simulink model "sgMdl_IO781_AFDXLoopback"  (R2024b)
settings: Solver=FixedStepAuto  StartTime=0.0  StopTime=inf  RelTol=1e-3  EnableMultiTasking=on
libraries: slrealtimeutilitieslib x4, speedgoatlib_IO781 x3, simulink x1
Description:
  | IO781 - AFDX Loopback
settings Model: sg_rtwmakecfg_data=_sg_IO75X_v1_2_0__a664api_  ModifiedByFormat=Speedgoat  SimulationMode=external  ExtModeTrigDuration=100000  Creator=Speedgoat  LastModifiedBy=Speedgoat
settings SolverCC: ConcurrentTasks=on  AlgebraicLoopSolver=TrustRegion  PositivePriorityOrder=on
settings DataIOCC: LimitDataPoints=on  SaveFormat=Array  ReturnWorkspaceOutputs=off
settings OptimizationCC: BlockReduction=off  OptimizeBlockIOStorage=off  BufferReuse=off  GlobalBufferReuse=off  ExpressionFolding=off  LocalBlockOutputs=off
settings DebuggingCC: UnderspecifiedInitializationDetection=Classic  MergeDetectMultiDrivingBlocksExec=none  SolverPrmCheckMsg=warning  TasksWithSamePriorityMsg=none  UnconnectedInputMsg=warning  UnconnectedOutputMsg=warning  UnconnectedLineMsg=warning  SFUnexpectedBacktrackingDiag=warning  SFNoUnconditionalDefaultTransitionDiag=warning  ArithmeticOperatorsInVariantConditions=warning
settings HardwareCC: ProdBitPerLong=64  ProdLongLongMode=on  ProdHWDeviceType=Intel->x86-64 (Linux 64)
settings ModelReferenceCC: EnableRefExpFcnMdlSchedulingChecks=on  PropagateSignalLabelsOutOfModel=off
settings SFSimCC: SimUseLocalCustomCode=off  CustomCodeUndefinedFunction=UseInterfaceOnly
settings RTWCC: Description=Speedgoat Real-Time Target Machine  SystemTargetFile=speedgoat.tlc  TemplateMakefile=slrealtime_default_tmf  RTWUseLocalCustomCode=off  Toolchain=Simulink Real-Time Toolchain  BuildConfiguration=Faster Runs  TargetLang=C++  GPUComputeCapability=3.5  DLArmComputeVersion=19.05
settings CodeAppCC: StateflowObjectComments=on
settings SimulinkRealTimeTargetCC: SubcomponentCodeInterfacePackaging=Reusable function  InstructionSetFMA=off  LogToMDFFile=off  SLRTFileLogMaxRuns=10  UseGCCFastMath=on
settings ConfigComp: CovMetricSettings=dw  CovSaveCumulativeToWorkspaceVar=on  CovSaveSingleToWorkspaceVar=on  CovExternalEMLEnable=off  CovSFcnEnable=off  CovBoundaryAbsTol=1.0e-5

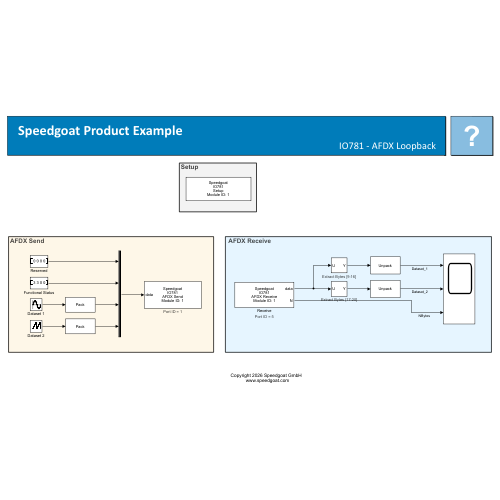
[thumbnail: Simulink's stored preview of the top-level diagram]
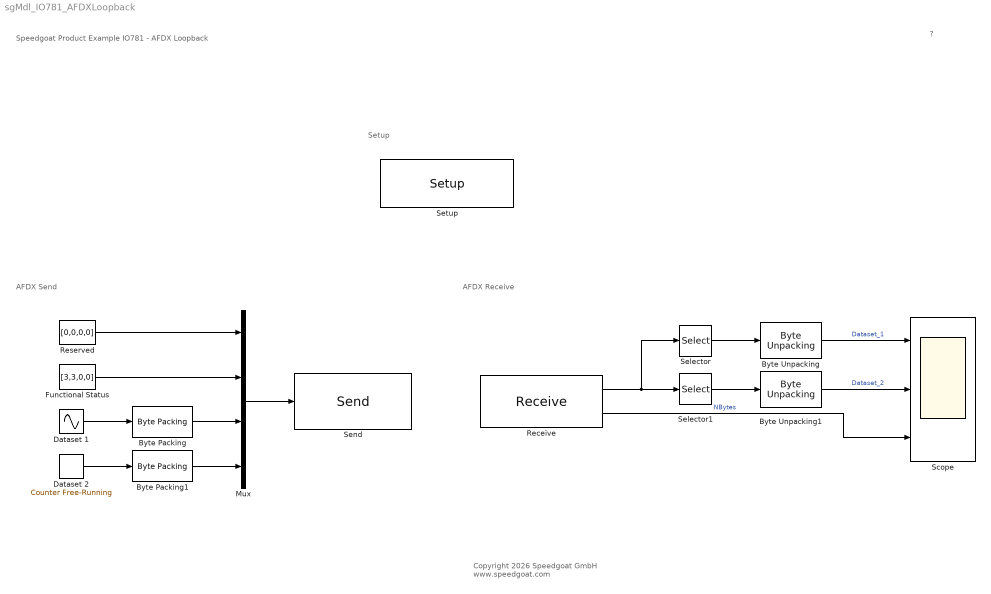
== system sgMdl_IO781_AFDXLoopback ==
  note: Setup
  note: AFDX Send
  note: AFDX Receive
  note: Speedgoat Product Example
      | IO781 - AFDX Loopback
  note: ?
  note: Copyright 2026 Speedgoat GmbH
      |  www.speedgoat.com
  Byte Packing : slrealtimeutilitieslib/Byte Packing  MaskPackedDataType=uint8  MaskUnpackedDataTypes={'double'}  MaskAlignment=1
  Byte Packing1 : slrealtimeutilitieslib/Byte Packing  MaskPackedDataType=uint8  MaskUnpackedDataTypes={'uint32'}  MaskAlignment=1
  Byte Unpacking : slrealtimeutilitieslib/Byte Unpacking  MaskUnpackedDataTypes={'double'}  MaskUnpackedDataSizes={[1]}  MaskAlignment=1
  Byte Unpacking1 : slrealtimeutilitieslib/Byte Unpacking  MaskUnpackedDataTypes={'uint32'}  MaskUnpackedDataSizes={[1]}  MaskAlignment=1
  Dataset 1 : Sin  Amplitude=50  Frequency=2*pi  SampleTime=0.01
  Dataset 2 : simulink/Sources/Counter Free-Running  NumBits=32  tsamp=0.01
  Functional Status : Constant  Value=[3,3,0,0]  OutDataTypeStr=uint8  SampleTime=0.01
  Mux : Mux
  Receive : speedgoatlib_IO781/Receive   parModuleId=1  parSampleTime=0.01  parPortId=5  parRxMsgLen=20
      settings: AttributesFormatString=Port ID = %<parPortId>  SourceProductName=Simulink Real-Time: Speedgoat Library
  "Reserved " : Constant  Value=[0,0,0,0]  OutDataTypeStr=uint8  SampleTime=0.01
  Scope : Scope  NumInputPorts=3
  Selector : Selector  InputPortWidth=20  IndexOptions=Index vector (dialog)  Indices=[9:16]  OutputSizes=1
      settings: AttributesFormatString=Extract Bytes %<Indices>
  Selector1 : Selector  InputPortWidth=20  IndexOptions=Index vector (dialog)  Indices=[17:20]  OutputSizes=1
      settings: AttributesFormatString=Extract Bytes %<Indices>
  "Send " : speedgoatlib_IO781/Send   parModuleId=1  parSampleTime=-1  parPortId=1  parTxMsgLen=20
      settings: AttributesFormatString=Port ID = %<parPortId>  SourceProductName=Simulink Real-Time: Speedgoat Library
  "Setup " : speedgoatlib_IO781/Setup   parModuleId=1  parConfigFile='IO781_Config.adc'
      settings: SourceProductName=Simulink Real-Time: Speedgoat Library
  wires:
  "Reserved "/1 -> Mux/1
  Functional Status/1 -> Mux/2
  Dataset 1/1 -> Byte Packing/1
  Mux/1 -> "Send "/1
  Byte Packing/1 -> Mux/3
  Receive/1 -> Selector1/1, Selector/1
  Byte Packing1/1 -> Mux/4
  Dataset 2/1 -> Byte Packing1/1
  Selector/1 -> Byte Unpacking/1
  Selector1/1 -> Byte Unpacking1/1
  Byte Unpacking1/1 -> Scope/2  "Dataset_2"
  Byte Unpacking/1 -> Scope/1  "Dataset_1"
  Receive/2 -> Scope/3  "NBytes"
